simulink model "neck_head_openloop_r2021b"  (R2021b)
settings: Solver=daessc  StartTime=0.0  StopTime=10  MaxStep=1e-3  RelTol=1e-3
model workspace (MAT data in the model file):
  Ts = 0.001
undefined symbols (not defined in the file): DCMotor, degrading_factors, front_pulley_diam, headData, roll_pitch_pid, side_pulley_diam, small_pulley_diam, smiData, timing_pulley_damping, timing_pulley_stiffness, torsional_filter_spring_stiffness, X, Y, yaw_pid, Z
libraries: sm_lib x1038, fl_lib x37, nesl_utility x31, slpidlib x3, ee_lib x3, sdl_lib x2, robotcorelib x1, simulink x1
(part 1 of 21)
settings Model: SimulationMode=accelerator  Creator=mfussi  LastModifiedBy=mfussi
settings DataIOCC: SaveOutput=off  DSMLogging=off  SaveTime=off
settings SimscapeCC: SimscapeLogLimitData=off  SimscapeCompileComponentReuse=on
settings DiagnosticsConfigSet: SimMechanicsUnconnectedFramePorts=none  SimMechanicsUnconnectedGeometryPorts=none
settings ExplorerConfigSet: InternalSimMechanicsExplorerSettings="<ExplorerConfiguration><canonicalview>default</canonicalview><AnimationSetting><BasePlaybackSpeed>1.0</BasePlaybackSpeed><PlaybackSpeedFactor>1.0</PlaybackSpeedFactor></AnimationSetting><TilePanel><TileInfo><Tiles Columns=\"2\" Count=\"2\" Rows=\"1\"><Column Weight=\"0.5\"/><Column Weight=\"0.5\"/><Row Weight=\"1\"/><Tile Height=\"1\" Width=\"1\" X=\"0\" Y=\"0\"/><Tile Height=\"1\" Width=\"1\" X=\"1\" Y=\"0\"/></Tiles></TileInfo><SceneInfo><SceneViewer><BGColor><R>1</R><G>1</G><B>1</B></BGColor><Camera><DoPerspective>off</DoPerspective><Position><X>0.609102614329787406</X><Y>0.611302486587517069</Y><Z>0.558963926748892614</Z></Position><Center><X>-0.0144419922031979002</X><Y>-0.0126323440951043794</Y><Z>0.0879040041013783857</Z></Center><Up><X>-0.356456120424211265</X><Y>-0.3093652744722587</Y><Z>0.881607713874387744</Z></Up><ViewLimDist>1</ViewLimDist><YLim>0.230031089988138981</YLim><XLim>0.18963268685469678</XLim></Camera></SceneViewer><SceneViewer><BGColor><R>1</R><G>1</G><B>1</B></BGColor><Camera><DoPerspective>off</DoPerspective><Position><X>0.00650661025794597829</X><Y>0.977869077349574845</Y><Z>0.103345502346217519</Z></Position><Center><X>0.00650661025794597829</X><Y>-0.0221309226504251555</Y><Z>0.103345502346217519</Z></Center><Up><X>0</X><Y>0</Y><Z>1</Z></Up><ViewLimDist>1</ViewLimDist><YLim>0.239000258580947006</YLim><XLim>0.197026676681005236</XLim></Camera></SceneViewer></SceneInfo></TilePanel><MechEditorPanel><Cameras/><GfxPanelCameraMap/><VideoCreator><PlaybackSpeedRatio>1.0</PlaybackSpeedRatio><FrameRate>30</FrameRate><VideoFormat>MPEG-4</VideoFormat><FrameSize>auto</FrameSize></VideoCreator></MechEditorPanel></ExplorerConfiguration>"

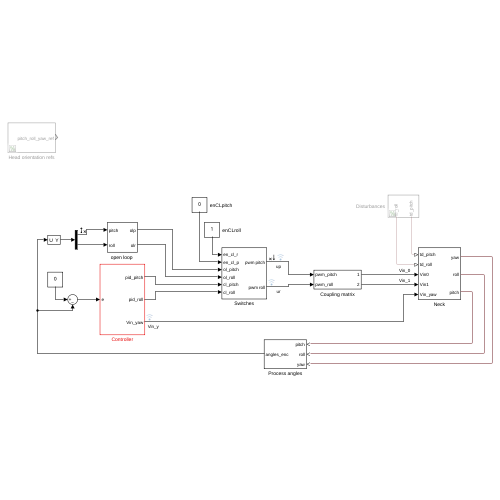
[thumbnail: Simulink's stored preview of the top-level diagram]
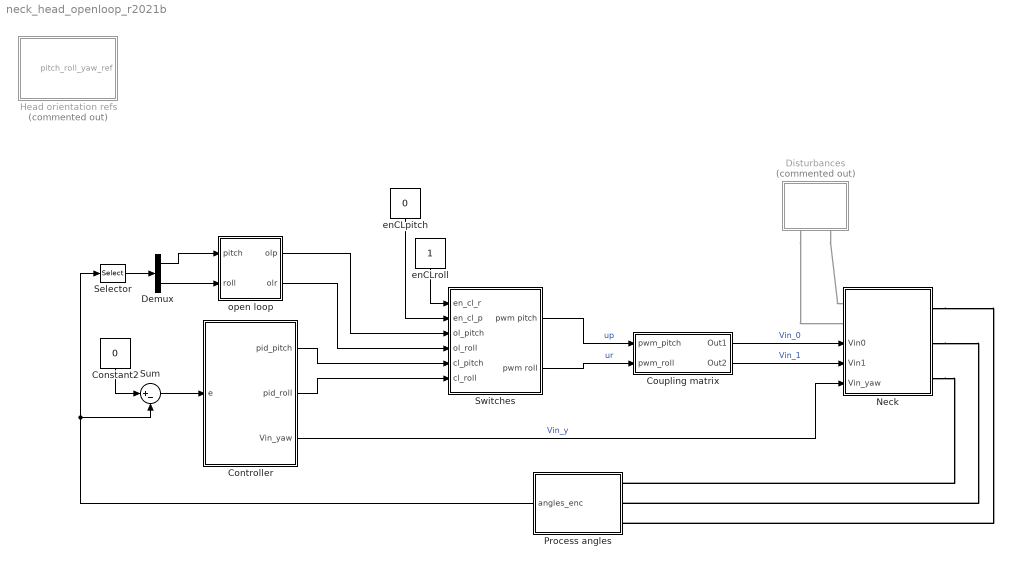
== system neck_head_openloop_r2021b ==
  Constant2 : Constant  Value=0
  Controller : Subsystem
  Coupling matrix : Subsystem
  Demux : Demux  Outputs=2
  Disturbances : Subsystem  Commented=on
  Head orientation refs : Subsystem  Commented=on
  Neck : Subsystem
      settings: PortSchema="{\"entries\":[{\"content\":{\"sides\":[{\"content\":{\"connectorIds\":[\"LConn1\",\"LConn2\",\"In1\",\"In2\",\"In3\"]},\"type\":\"ConnectorPlacement.EquallySpacedRectSide\",\"uuid\":\"f7883834-26e2-4ef8-86bb-9a9befb8627d\"},{\"content\":{\"connectorIds\":[\"RConn1\",\"RConn2\",\"RConn3\"],\"side\":\"RIGHT\"},\"type\":\"ConnectorPlacement.EquallySpacedRectSide\",\"uuid\":\"9cd534f4-893a-4016-87b9-a61185e18a66\"},{\"content\":{\"connectorIds\":[],\"side\":\"TOP\"},\"type\":\"ConnectorPlacement.EquallySpacedRectSide\",\"uuid\":\"6ed62664-4466-4c61-883e-9679ae4c4566\"}]},\"type\":\"ConnectorPlacement.EquallySpacedConnector\",\"uuid\":\"47674466-cec6-46c2-a828-d70cf59b2873\"}],\"packageUris\":[\"http://schema.mathworks.com/mf0/Connector/R2020b\"],\"version\":\"1.0\"}"
  Process angles : Subsystem
  Selector : Selector  InputPortWidth=3  IndexOptions=Index vector (dialog)  Indices=[1 2]  OutputSizes=1
  Sum : Sum  Inputs=|+-
  Switches : Subsystem
  enCLpitch : Constant  Value=0
  enCLroll : Constant
  "open loop " : Subsystem
  wires:
  Controller/3(Vin_yaw) -> Neck/3(Vin_yaw)  "Vin_y"
  Coupling matrix/2(Out2) -> Neck/2(Vin1)  "Vin_1"
  Sum/1 -> Controller/1(e)
  Coupling matrix/1(Out1) -> Neck/1(Vin0)  "Vin_0"
  Constant2/1 -> Sum/1
  enCLpitch/1 -> Switches/2(en_cl_p)
  enCLroll/1 -> Switches/1(en_cl_r)
  Controller/1(pid_pitch) -> Switches/5(cl_pitch)
  Controller/2(pid_roll) -> Switches/6(cl_roll)
  Switches/1(pwm pitch) -> Coupling matrix/1(pwm_pitch)  "up"
  Switches/2(pwm roll) -> Coupling matrix/2(pwm_roll)  "ur"
  "open loop "/1(olp) -> Switches/3(ol_pitch)
  "open loop "/2(olr) -> Switches/4(ol_roll)
  Demux/1 -> "open loop "/1(pitch)
  Demux/2 -> "open loop "/2(roll)
  Process angles/1(angles_enc) -> Selector/1, Sum/2
  Selector/1 -> Demux/1
  connections:
  Neck/RConn1 -- Process angles/LConn3
  Neck/RConn2 -- Process angles/LConn2
  Neck/RConn3 -- Process angles/LConn1
  Disturbances/RConn2 -- Neck/LConn1
  Disturbances/RConn1 -- Neck/LConn2

== system neck_head_openloop_r2021b/Controller ==
  e : Inport
  Demux : Demux  Outputs=3
  Discrete PID Controller : slpidlib/PID Controller  Controller=PID  Form=Parallel  TimeDomain=Discrete-time  UseExternalTs=off  SampleTime=Ts  IntegratorMethod=Trapezoidal  FilterMethod=Trapezoidal  ControllerParametersSource=internal  P=roll_pitch_pid.p * degrading_factors.pid_detune  I=roll_pitch_pid.i * degrading_factors.pid_detune  D=roll_pitch_pid.d * degrading_factors.pid_detune  N=roll_pitch_pid.n * degrading_factors.pid_detune  UseFilter=on  TunerSelectOption=Transfer Function Based (PID Tuner App)  InitialConditionSource=internal  InitialConditionForIntegrator=0  InitialConditionForFilter=0  DifferentiatorICPrevScaledInput=0  ExternalReset=none  TrackingMode=off  Kt=1  LimitOutput=on  SatLimitsSource=internal  UpperSaturationLimit=roll_pitch_pid.u_max  LowerSaturationLimit=roll_pitch_pid.u_min  LinearizeAsGain=off  AntiWindupMode=back-calculation  Kb=roll_pitch_pid.i  POutMin=[]  POutMax=[]  IOutMin=[]  IOutMax=[]  DOutMin=[]  DOutMax=[]  NOutMin=[]  NOutMax=[]  SumOutMin=[]  SumOutMax=[]  SaturationOutMin=[]  SaturationOutMax=[]  PParamMin=[]  PParamMax=[]  IParamMin=[]  IParamMax=[]  DParamMin=[]  DParamMax=[]  NParamMin=[]  NParamMax=[]  KbParamMin=[]  KbParamMax=[]  KtParamMin=[]  KtParamMax=[]  KbOutMin=[]  KbOutMax=[]  KtOutMin=[]  KtOutMax=[]  IntegratorOutMin=[]  IntegratorOutMax=[]  FilterOutMin=[]  FilterOutMax=[]  SumI1OutMin=[]  SumI1OutMax=[]  SumI2OutMin=[]  SumI2OutMax=[]  SumI3OutMin=[]  SumI3OutMax=[]  SumI4OutMin=[]  SumI4OutMax=[]  SumDOutMin=[]  SumDOutMax=[]  DifferentiatorOutMin=[]  DifferentiatorOutMax=[]  FilterDiffOutCoefMin=[]  FilterDiffOutCoefMax=[]  ReciprocalOutMin=[]  ReciprocalOutMax=[]  SumDenOutMin=[]  SumDenOutMax=[]  SumNumOutMin=[]  SumNumOutMax=[]  DivideOutMin=[]  DivideOutMax=[]  UdiffTsProdOutMin=[]  UdiffTsProdOutMax=[]  NTsProdOutMin=[]  NTsProdOutMax=[]  UintegralTsProdOutMin=[]  UintegralTsProdOutMax=[]  UngainTsProdOutMin=[]  UngainTsProdOutMax=[]  IntegratorContinuousStateAttributes=''  IntegratorStateMustResolveToSignalObject=off  IntegratorRTWStateStorageClass=Auto  FilterContinuousStateAttributes=''  FilterStateMustResolveToSignalObject=off  FilterRTWStateStorageClass=Auto  ParallelPVariant=InternalParameters  IdealPVariant=Disabled  IVariant=InternalParameters  DVariant=InternalParameters  IntegratorVariant=Discrete  SatVariant=Enabled  AWVariant=BackCalculation  PCopyVariant=Disabled  TRVariant=Disabled  FdbkBlocksVariant=Feedback  IdealPFdbkVariant=Passthrough  SatFdbkVariant=Enabled  DerivativeFilterVariant=TrapezoidalFilter  NVariant=InternalParameters  NCopyVariant=InternalParameters  FilterICVariant=InternalICsFilter  IntegratorICVariant=InternalICs  ExternalResetVariant=Disabled  TRSumVariant=Passthrough  SumFdbkVariant=Enabled  SumVariant=Sum_PID  TsampFilterVariant=InternalTs  TsampNgainVariant=Passthrough  TsampIntegralVariant=Passthrough  ExternalSaturationOutDataTypeStr=Inherit: Same as second input
  Discrete PID Controller1 : slpidlib/PID Controller  Controller=PID  Form=Parallel  TimeDomain=Discrete-time  UseExternalTs=off  SampleTime=Ts  IntegratorMethod=Trapezoidal  FilterMethod=Trapezoidal  ControllerParametersSource=internal  P=roll_pitch_pid.p * degrading_factors.pid_detune  I=roll_pitch_pid.i * degrading_factors.pid_detune  D=roll_pitch_pid.d * degrading_factors.pid_detune  N=roll_pitch_pid.n * degrading_factors.pid_detune  UseFilter=on  TunerSelectOption=Transfer Function Based (PID Tuner App)  InitialConditionSource=internal  InitialConditionForIntegrator=0  InitialConditionForFilter=0  DifferentiatorICPrevScaledInput=0  ExternalReset=none  TrackingMode=off  Kt=1  LimitOutput=on  SatLimitsSource=internal  UpperSaturationLimit=roll_pitch_pid.u_max  LowerSaturationLimit=roll_pitch_pid.u_min  LinearizeAsGain=off  AntiWindupMode=back-calculation  Kb=roll_pitch_pid.i  POutMin=[]  POutMax=[]  IOutMin=[]  IOutMax=[]  DOutMin=[]  DOutMax=[]  NOutMin=[]  NOutMax=[]  SumOutMin=[]  SumOutMax=[]  SaturationOutMin=[]  SaturationOutMax=[]  PParamMin=[]  PParamMax=[]  IParamMin=[]  IParamMax=[]  DParamMin=[]  DParamMax=[]  NParamMin=[]  NParamMax=[]  KbParamMin=[]  KbParamMax=[]  KtParamMin=[]  KtParamMax=[]  KbOutMin=[]  KbOutMax=[]  KtOutMin=[]  KtOutMax=[]  IntegratorOutMin=[]  IntegratorOutMax=[]  FilterOutMin=[]  FilterOutMax=[]  SumI1OutMin=[]  SumI1OutMax=[]  SumI2OutMin=[]  SumI2OutMax=[]  SumI3OutMin=[]  SumI3OutMax=[]  SumI4OutMin=[]  SumI4OutMax=[]  SumDOutMin=[]  SumDOutMax=[]  DifferentiatorOutMin=[]  DifferentiatorOutMax=[]  FilterDiffOutCoefMin=[]  FilterDiffOutCoefMax=[]  ReciprocalOutMin=[]  ReciprocalOutMax=[]  SumDenOutMin=[]  SumDenOutMax=[]  SumNumOutMin=[]  SumNumOutMax=[]  DivideOutMin=[]  DivideOutMax=[]  UdiffTsProdOutMin=[]  UdiffTsProdOutMax=[]  NTsProdOutMin=[]  NTsProdOutMax=[]  UintegralTsProdOutMin=[]  UintegralTsProdOutMax=[]  UngainTsProdOutMin=[]  UngainTsProdOutMax=[]  IntegratorContinuousStateAttributes=''  IntegratorStateMustResolveToSignalObject=off  IntegratorRTWStateStorageClass=Auto  FilterContinuousStateAttributes=''  FilterStateMustResolveToSignalObject=off  FilterRTWStateStorageClass=Auto  ParallelPVariant=InternalParameters  IdealPVariant=Disabled  IVariant=InternalParameters  DVariant=InternalParameters  IntegratorVariant=Discrete  SatVariant=Enabled  AWVariant=BackCalculation  PCopyVariant=Disabled  TRVariant=Disabled  FdbkBlocksVariant=Feedback  IdealPFdbkVariant=Passthrough  SatFdbkVariant=Enabled  DerivativeFilterVariant=TrapezoidalFilter  NVariant=InternalParameters  NCopyVariant=InternalParameters  FilterICVariant=InternalICsFilter  IntegratorICVariant=InternalICs  ExternalResetVariant=Disabled  TRSumVariant=Passthrough  SumFdbkVariant=Enabled  SumVariant=Sum_PID  TsampFilterVariant=InternalTs  TsampNgainVariant=Passthrough  TsampIntegralVariant=Passthrough  ExternalSaturationOutDataTypeStr=Inherit: Same as second input
  Discrete PID Controller2 : slpidlib/PID Controller  Controller=PI  Form=Parallel  TimeDomain=Discrete-time  UseExternalTs=off  SampleTime=Ts  IntegratorMethod=Trapezoidal  FilterMethod=Trapezoidal  ControllerParametersSource=internal  P=yaw_pid.p  I=yaw_pid.i  D=0  N=1011.6661131708  UseFilter=on  TunerSelectOption=Transfer Function Based (PID Tuner App)  InitialConditionSource=internal  InitialConditionForIntegrator=0  InitialConditionForFilter=0  DifferentiatorICPrevScaledInput=0  ExternalReset=none  TrackingMode=off  Kt=1  LimitOutput=on  SatLimitsSource=internal  UpperSaturationLimit=yaw_pid.u_max  LowerSaturationLimit=yaw_pid.u_min  LinearizeAsGain=off  AntiWindupMode=back-calculation  Kb=yaw_pid.i  POutMin=[]  POutMax=[]  IOutMin=[]  IOutMax=[]  DOutMin=[]  DOutMax=[]  NOutMin=[]  NOutMax=[]  SumOutMin=[]  SumOutMax=[]  SaturationOutMin=[]  SaturationOutMax=[]  PParamMin=[]  PParamMax=[]  IParamMin=[]  IParamMax=[]  DParamMin=[]  DParamMax=[]  NParamMin=[]  NParamMax=[]  KbParamMin=[]  KbParamMax=[]  KtParamMin=[]  KtParamMax=[]  KbOutMin=[]  KbOutMax=[]  KtOutMin=[]  KtOutMax=[]  IntegratorOutMin=[]  IntegratorOutMax=[]  FilterOutMin=[]  FilterOutMax=[]  SumI1OutMin=[]  SumI1OutMax=[]  SumI2OutMin=[]  SumI2OutMax=[]  SumI3OutMin=[]  SumI3OutMax=[]  SumI4OutMin=[]  SumI4OutMax=[]  SumDOutMin=[]  SumDOutMax=[]  DifferentiatorOutMin=[]  DifferentiatorOutMax=[]  FilterDiffOutCoefMin=[]  FilterDiffOutCoefMax=[]  ReciprocalOutMin=[]  ReciprocalOutMax=[]  SumDenOutMin=[]  SumDenOutMax=[]  SumNumOutMin=[]  SumNumOutMax=[]  DivideOutMin=[]  DivideOutMax=[]  UdiffTsProdOutMin=[]  UdiffTsProdOutMax=[]  NTsProdOutMin=[]  NTsProdOutMax=[]  UintegralTsProdOutMin=[]  UintegralTsProdOutMax=[]  UngainTsProdOutMin=[]  UngainTsProdOutMax=[]  IntegratorContinuousStateAttributes=''  IntegratorStateMustResolveToSignalObject=off  IntegratorRTWStateStorageClass=Auto  FilterContinuousStateAttributes=''  FilterStateMustResolveToSignalObject=off  FilterRTWStateStorageClass=Auto  ParallelPVariant=InternalParameters  IdealPVariant=Disabled  IVariant=InternalParameters  DVariant=Disabled  IntegratorVariant=Discrete  SatVariant=Enabled  AWVariant=BackCalculation  PCopyVariant=Disabled  TRVariant=Disabled  FdbkBlocksVariant=Feedback  IdealPFdbkVariant=Passthrough  SatFdbkVariant=Enabled  DerivativeFilterVariant=Disabled  NVariant=Disabled  NCopyVariant=Disabled_SignalSpec  FilterICVariant=Disabled  IntegratorICVariant=InternalICs  ExternalResetVariant=Disabled  TRSumVariant=Passthrough  SumFdbkVariant=Enabled  SumVariant=Sum_PI  TsampFilterVariant=InternalTs  TsampNgainVariant=Passthrough  TsampIntegralVariant=Passthrough  ExternalSaturationOutDataTypeStr=Inherit: Same as second input
  pid_pitch : Outport
  pid_roll : Outport  Port=2
  Vin_yaw : Outport  Port=3
  wires:
  Discrete PID Controller2/1 -> Vin_yaw/1
  e/1 -> Demux/1  "e"
  Discrete PID Controller/1 -> pid_pitch/1  "pid_pitch"
  Demux/3 -> Discrete PID Controller2/1  "e_yaw"
  Demux/2 -> Discrete PID Controller1/1  "e_roll"
  Discrete PID Controller1/1 -> pid_roll/1  "pid_roll"
  Demux/1 -> Discrete PID Controller/1  "e_pitch"

== system neck_head_openloop_r2021b/Coupling matrix ==
  pwm_pitch : Inport
  pwm_roll : Inport  Port=2
  Sum1 : Sum  Inputs=|++
  Sum4 : Sum  Inputs=-+|
  Out1 : Outport
  Out2 : Outport  Port=2
  wires:
  Sum1/1 -> Out1/1
  pwm_roll/1 -> Sum4/2, Sum1/2
  pwm_pitch/1 -> Sum4/1, Sum1/1
  Sum4/1 -> Out2/1

== system neck_head_openloop_r2021b/Disturbances ==
  Add : Sum
  Add1 : Sum
  Constant : Constant  Value=smiData.RevoluteJoint(3).Rz.Pos
  Constant1 : Constant  Value=smiData.RevoluteJoint(6).Rz.Pos
  Disturbance trigger : Step  SampleTime=0
  Mux : Mux  Inputs=2
  Product : Product
  Product1 : Product
  Simulink-PS Converter : nesl_utility/Simulink-PS Converter  PhysicalDomain=network_engine_domain  SubClassName=ps_input  LeftPortType=input  RightPortType=output  PseudoPeriodic=off  Frequencies=[]  NoiseDistribution=none  NoiseParameters=[]  Unit=deg  AffineConversion=off  FilteringAndDerivatives=filter  SimscapeFilterOrder=2  InputFilterTimeConstant=0.001  UdotUserProvided=0
      settings: SourceProductBaseCode=SS,PW,VE
  Simulink-PS Converter1 : nesl_utility/Simulink-PS Converter  PhysicalDomain=network_engine_domain  SubClassName=ps_input  LeftPortType=input  RightPortType=output  PseudoPeriodic=off  Frequencies=[]  NoiseDistribution=none  NoiseParameters=[]  Unit=deg  AffineConversion=off  FilteringAndDerivatives=filter  SimscapeFilterOrder=2  InputFilterTimeConstant=0.001  UdotUserProvided=0
      settings: SourceProductBaseCode=SS,PW,VE
  To Workspace : ToWorkspace  VariableName=disturbances  SaveFormat=Timeseries  SampleTime=-1
  pitch disturbance : Sin  Amplitude=0.2  Frequency=3 / 2* pi  SampleTime=0
  roll disturbance : Sin  Amplitude=0.2  Frequency=3 / 2* pi  SampleTime=0
  td_roll : PMIOPort  Side=Right
  td_pitch : PMIOPort  Port=2  Side=Right
  wires:
  pitch disturbance/1 -> Product/1
  Disturbance trigger/1 -> Product1/1, Product/2
  roll disturbance/1 -> Product1/2
  Mux/1 -> To Workspace/1
  Product/1 -> Add/2
  Product1/1 -> Add1/1
  Add1/1 -> Mux/2, Simulink-PS Converter1/1
  Constant/1 -> Add/1
  Constant1/1 -> Add1/2
  Add/1 -> Mux/1, Simulink-PS Converter/1
  connections:
  td_pitch/RConn1 -- Simulink-PS Converter/RConn1
  td_roll/RConn1 -- Simulink-PS Converter1/RConn1

== system neck_head_openloop_r2021b/Head orientation refs ==
  Min-jerk roll pitch references : robotcorelib/Polynomial Trajectory  WaypointSource=Internal  Waypoints=wp  TimePoints=tp  TimeInterval=[ 1, 4 ]  Method=Quintic Polynomial  ParameterSource=Internal  VelocityBoundaryCondition=vel_bounds  AccelerationBoundaryCondition=accel_bounds  SimulateUsing=Code generation
      settings: SourceProductBaseCode=RO,NV,RR,UV
  Mux : Mux  Inputs=2
  Ramp : simulink/Sources/Ramp  slope=1  start=0  InitialOutput=0
  Terminator : Terminator
  Terminator1 : Terminator
  To Workspace : ToWorkspace  VariableName=ref  SaveFormat=Timeseries  SampleTime=-1
  Zero-Order Hold : ZeroOrderHold  SampleTime=-1
  yaw reference : Constant  Value=0
  pitch_roll_yaw_ref : Outport
  wires:
  Min-jerk roll pitch references/3 -> Terminator1/1
  Min-jerk roll pitch references/1 -> Mux/1
  Min-jerk roll pitch references/2 -> Terminator/1
  Ramp/1 -> Zero-Order Hold/1
  Zero-Order Hold/1 -> Min-jerk roll pitch references/1
  yaw reference/1 -> Mux/2
  Mux/1 -> To Workspace/1, pitch_roll_yaw_ref/1  "p-r-y ref"
